simulink library "myLibrary"  (R2015b)
settings: Solver=VariableStepAuto  StartTime=0.0  StopTime=10.0  RelTol=1e-3
values from neighbouring files (symbols this model uses):
  adapt = 1    [init.m]    (also in init_model.m; init_mussels.m; init_mussels_2.m; init_mussels_konfiguracija_blizu.m)
  sigma_0 = [ 0    0.7   0    0    0 ... (first row only)    [init.m]    (also in init_model.m = zeros(M,M); init_mussels.m = zeros(n,n); init_mussels_2.m; init_mussels_konfiguracija_blizu.m = [ 0    0.7   0.4    0.6    0.5)
  zeta_0 = zeros(n,n)    [init.m]    (also in init_model.m = zeros(M,M); init_mussels.m; init_mussels_2.m; init_mussels_konfiguracija_blizu.m)
settings Model: Creator=Tamara  LastModifiedBy=Tamara

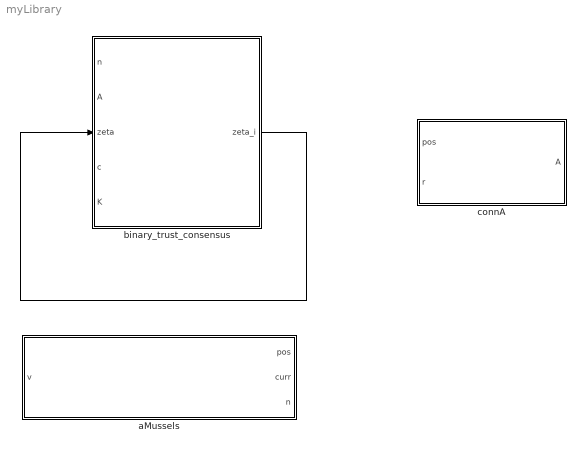
== system myLibrary ==
  aMussels : Subsystem
  "binary_trust_consensus " : Subsystem
  connA : MATLAB Function  TreatAsAtomicUnit=on
  wires:
  "binary_trust_consensus "/1(zeta_i) -> "binary_trust_consensus "/3(zeta)

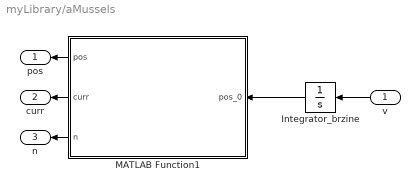
== system myLibrary/aMussels ==
  v : Inport
  Integrator_brzine : Integrator  InitialCondition=[0 0 0 0 0;0 0 0 0 0;0 0 0 0 0]
  MATLAB Function1 : MATLAB Function  TreatAsAtomicUnit=on
  pos : Outport
  curr : Outport  Port=2
  n : Outport  Port=3
  wires:
  Integrator_brzine/1 -> MATLAB Function1/1(pos_0)
  MATLAB Function1/3(n) -> n/1
  MATLAB Function1/2(curr) -> curr/1
  v/1 -> Integrator_brzine/1
  MATLAB Function1/1(pos) -> pos/1

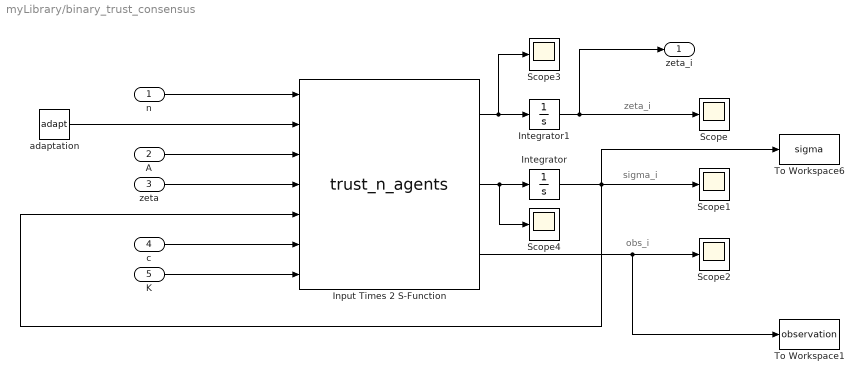
== system myLibrary/binary_trust_consensus  ==
  note: obs_i
  note: sigma_i
  note: zeta_i
  n : Inport
  A : Inport  Port=2
  zeta : Inport  Port=3
  c : Inport  Port=4
  K : Inport  Port=5
  Input Times 2 S-Function : S-Function  FunctionName=trust_n_agents  SFunctionDeploymentMode=off  EnableBusSupport=off
  Integrator : Integrator  InitialCondition=sigma_0
  Integrator1 : Integrator  InitialCondition=zeta_0
  Scope{,1..4} (5 alike) : Scope
  To Workspace1 : ToWorkspace  VariableName=observation  SampleTime=-1
  To Workspace6 : ToWorkspace  VariableName=sigma  SampleTime=-1
  adaptation : Constant  Value=adapt
  zeta_i : Outport
  wires:
  Integrator/1 -> Input Times 2 S-Function/5, To Workspace6/1, Scope1/1
  Integrator1/1 -> zeta_i/1, Scope/1
  c/1 -> Input Times 2 S-Function/6
  K/1 -> Input Times 2 S-Function/7
  Input Times 2 S-Function/2 -> Scope4/1, Integrator/1
  Input Times 2 S-Function/1 -> Scope3/1, Integrator1/1
  Input Times 2 S-Function/3 -> To Workspace1/1, Scope2/1
  n/1 -> Input Times 2 S-Function/1
  adaptation/1 -> Input Times 2 S-Function/2
  zeta/1 -> Input Times 2 S-Function/4
  A/1 -> Input Times 2 S-Function/3

== matlab function myLibrary/connA ==
  data: pos input; r input; A output
function A  = scenario(pos, r)
%#codegen
%radijus komunikacije
%r = 0.01;

n=length(pos);
%[m,n] = size(pos);
%inicijalizacija matrice A
A=zeros(n);

for i = 1:n
    for j = 1:n
        %odredivanje udaljenosti izmedju musula - prvo x, y, pa z
        distance = sqrt((pos(1,i)-pos(1,j))^2 + (pos(2,i)-pos(2,j))^2+(pos(3,i)-pos(3,j))^2);
        
        %provjera mogu li komunicirati
        if distance < r
            
            %element ne komunicira sam sa sobom
            if i == j
                A(i,j) = 0;
            else
                A(i,j) = 1;
            end
                        
        else
            A(i,j) = 0;
        end
        
    end
       
end


end

== matlab function myLibrary/aMussels/MATLAB Function1 ==
  data: pos output; curr output; n output; pos_0 input
function [pos, curr, n] = mussels (pos_0)
%#codegen
%u inpute bi trebalo dodati koordinate, deltu i zetu?

n=5;
pos = pos_0;

X = zeros(1,n);
Y = zeros(1,n);
Z = zeros(1,n);

%mussels su blizu jedna druge
%{
X(1) = 1;
Y(1) = 1;
Z = zeros(1,n);

for i = 2 : n
    
    X(i) = X(i-1)+0.1;
    Y(i) = Y(i-1)+0.1;

end
%}
%mussels su rasprsene


X(1) = 1;
Y(1) = 1;
Z = zeros(1,n);

for i = 2 : n
    
    X(i) = X(i-1)+10;
    Y(i) = Y(i-1)+10;

end


%{
%random postavljanje koordinata
X = randperm(15,n); 
Y = randperm(15,n);
Z = zeros(1,n);
%}

%stvaranje matrice pozicije
    pos(1,:) = X;
    pos(2,:) = Y;
    pos(3,:) = Z;

%mjerenja
curr = randi(3,size(X));

end
